simulink library "HIL_GenSet"  (Simulink 7.8)
settings: Solver=ode45  StartTime=0.0  StopTime=10.0  RelTol=1e-3
values from neighbouring files (symbols this model uses):
  Ts = 80e-6    (= 8e-05)    [global_parameters.m]    (also in scopeBuffer.m)
undefined symbols (not defined in the file or in its folder): DiscIntNeverNeededParam, Ts_Power
libraries: simulink x77, powerlib x55, discretizing x28
(part 1 of 9)
settings Model: Creator=RE25624  LastModifiedBy=re25624

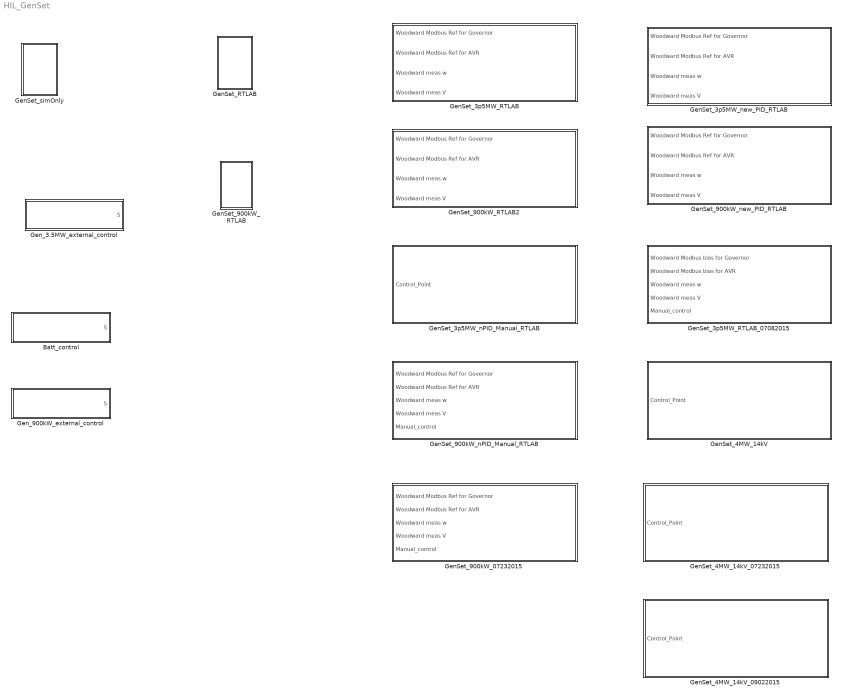
== system HIL_GenSet ==
  Batt_control : Subsystem
  GenSet_3p5MW_RTLAB : Subsystem  mask(Gen-Set with simulated control modes){mode=1 (PQ), set_Pref=0.8, set_Qref=.5, set_vref=1, set_wref=1, enable_gen=1, control_mode=0}
      mask prompts: set_Pref "Active power reference [p.u.]"; set_Qref "Reactive power reference [p.u.]"; set_vref "Terminal voltage reference [p.u.]"; set_wref "Frequency reference [p.u.]"; enable_gen "Enable generator"; control_mode "Control Mode [0 => Sim. 1 => Wood.]"
      mask help:
      | This Gen-Set block allows the user to indicate the control mode of the generator. The available control modes are: (1) PQ, (2) PV, and (3) VF.
      | The input values to the block will be applied according to the selected control mode.
      | For example, if PQ mode is selected, the controller will only work based on P_ref and Q_ref ignoring values of other inputs to the block.
      | *** This model will not interface with a hardware controller ***
      mask StyleString: popup(1 (PQ)|2 (PV)|3 (VF)),edit,edit,edit,edit,popup(1|0),edit
  GenSet_3p5MW_RTLAB_07082015 : Subsystem  mask(Gen-Set (3.5MW) with simulated control modes){control_mode=0}
      mask prompts: control_mode "Control Mode [0 => Sim. 1 => Wood.]"
      mask help:
      | This Gen-Set block (3.5MW) allows the user to indicate the control mode of the generator. The available control modes are: (1) PQ, (2) PV, and (3) VF.
      | The input values to the block will be applied according to the selected control mode.
      | For example, if PQ mode is selected, the controller will only work based on P_ref and Q_ref ignoring values of other inputs to the block.
      | *** This model will not interface with a hardware controller ***
  GenSet_3p5MW_nPID_Manual_RTLAB : Subsystem
      mask Type: Gen-Set (3.5MW) with simulated control modes
      mask Description:
      | This Gen-Set block (3.5MW) allows the user to indicate the control mode of the generator. The available control modes are: (1) PQ, (2) PV, and (3) VF.
      | The input values to the block will be applied according to the selected control mode.
      | For example, if PQ mode is selected, the controller will only work based on P_ref and Q_ref ignoring values of other inputs to the block.
      | *** This model will not interface with a hardware controller ***
      | 
      | Input parameters (as per unit of rated power):
      | P[p.u]: real power
      | Q[p.u]: reactive power
      | V[p.u]: voltage
      | F[p.u]: frequency
      | Mode: (1) PQ, (2) PV, and (3) VF.
  GenSet_3p5MW_new_PID_RTLAB : Subsystem  mask(Gen-Set with simulated control modes){mode=1 (PQ), set_Pref=0.8, set_Qref=0.2, set_vref=1, set_wref=1, enable_gen=1, control_mode=0}
      mask prompts: set_Pref "Active power reference [p.u.]"; set_Qref "Reactive power reference [p.u.]"; set_vref "Terminal voltage reference [p.u.]"; set_wref "Frequency reference [p.u.]"; enable_gen "Enable generator"; control_mode "Control Mode [0 => Sim. 1 => Wood.]"
      mask help:
      | This Gen-Set block allows the user to indicate the control mode of the generator. The available control modes are: (1) PQ, (2) PV, and (3) VF.
      | The input values to the block will be applied according to the selected control mode.
      | For example, if PQ mode is selected, the controller will only work based on P_ref and Q_ref ignoring values of other inputs to the block.
      | *** This model will not interface with a hardware controller ***
      mask StyleString: popup(1 (PQ)|2 (PV)|3 (VF)),edit,edit,edit,edit,popup(1|0),edit
  GenSet_4MW_14kV : Subsystem
      mask Type: Gen-Set (3.5MW) with simulated control modes
      mask Description:
      | This Gen-Set block (3.5MW) allows the user to indicate the control mode of the generator. The available control modes are: (1) PQ, (2) PV, and (3) VF.
      | The input values to the block will be applied according to the selected control mode.
      | For example, if PQ mode is selected, the controller will only work based on P_ref and Q_ref ignoring values of other inputs to the block.
      | *** This model will not interface with a hardware controller ***
      | 
      | Input parameters (as per unit of rated power):
      | P[p.u]: real power
      | Q[p.u]: reactive power
      | V[p.u]: voltage
      | F[p.u]: frequency
      | Mode: (1) PQ, (2) PV, and (3) VF.
  GenSet_4MW_14kV_07232015 : Subsystem
      mask Type: Gen-Set (3.5MW) with simulated control modes
      mask Description:
      | This Gen-Set block (3.5MW) allows the user to indicate the control mode of the generator. The available control modes are: (1) PQ, (2) PV, and (3) VF.
      | The input values to the block will be applied according to the selected control mode.
      | For example, if PQ mode is selected, the controller will only work based on P_ref and Q_ref ignoring values of other inputs to the block.
      | *** This model will not interface with a hardware controller ***
      | 
      | Input parameters (as per unit of rated power):
      | P[p.u]: real power
      | Q[p.u]: reactive power
      | V[p.u]: voltage
      | F[p.u]: frequency
      | Mode: (1) PQ, (2) PV, and (3) VF.
  GenSet_4MW_14kV_09022015 : Subsystem
      mask Type: Gen-Set (3.5MW) with simulated control modes
      mask Description:
      | This Gen-Set block (3.5MW) allows the user to indicate the control mode of the generator. The available control modes are: (1) PQ, (2) PV, and (3) VF.
      | The input values to the block will be applied according to the selected control mode.
      | For example, if PQ mode is selected, the controller will only work based on P_ref and Q_ref ignoring values of other inputs to the block.
      | *** This model will not interface with a hardware controller ***
      | 
      | Input parameters (as per unit of rated power):
      | P[p.u]: real power
      | Q[p.u]: reactive power
      | V[p.u]: voltage
      | F[p.u]: frequency
      | Mode: (1) PQ, (2) PV, and (3) VF.
  GenSet_900kW_07232015 : Subsystem  mask(Gen-Set with simulated control modes){control_mode=0}
      mask prompts: control_mode "Control Mode [0 => Sim. 1 => Wood.]"
      mask help:
      | This Gen-Set block allows the user to indicate the control mode of the generator. The available control modes are: (1) PQ, (2) PV, and (3) VF.
      | The input values to the block will be applied according to the selected control mode.
      | For example, if PQ mode is selected, the controller will only work based on P_ref and Q_ref ignoring values of other inputs to the block.
  GenSet_900kW_RTLAB : Subsystem  mask(Gen-Set with simulated control modes){mode=1 (PQ), set_Pref=0.95, set_Qref=0.85, set_vref=1, set_wref=1, enable_gen=1}
      mask prompts: set_Pref "Active power reference [p.u.]"; set_Qref "Reactive power reference [p.u.]"; set_vref "Terminal voltage reference [p.u.]"; set_wref "Frequency reference [p.u.]"; enable_gen "Enable generator"
      mask help:
      | This Gen-Set block allows the user to indicate the control mode of the generator. The available control modes are: (1) PQ, (2) PV, and (3) VF.
      | The input values to the block will be applied according to the selected control mode.
      | For example, if PQ mode is selected, the controller will only work based on P_ref and Q_ref ignoring values of other inputs to the block.
      | *** This model will not interface with a hardware controller ***
      mask StyleString: popup(1 (PQ)|2 (PV)|3 (VF)),edit,edit,edit,edit,popup(1|0)
  GenSet_900kW_RTLAB2 : Subsystem  mask(Gen-Set with simulated control modes){mode=1 (PQ), set_Pref=0.8, set_Qref=0.2, set_vref=1, set_wref=1, enable_gen=1, control_mode=0}
      mask prompts: set_Pref "Active power reference [p.u.]"; set_Qref "Reactive power reference [p.u.]"; set_vref "Terminal voltage reference [p.u.]"; set_wref "Frequency reference [p.u.]"; enable_gen "Enable generator"; control_mode "Control Mode [0 => Sim. 1 => Wood.]"
      mask help:
      | This Gen-Set block allows the user to indicate the control mode of the generator. The available control modes are: (1) PQ, (2) PV, and (3) VF.
      | The input values to the block will be applied according to the selected control mode.
      | For example, if PQ mode is selected, the controller will only work based on P_ref and Q_ref ignoring values of other inputs to the block.
      | *** This model will not interface with a hardware controller ***
      mask StyleString: popup(1 (PQ)|2 (PV)|3 (VF)),edit,edit,edit,edit,popup(1|0),edit
  GenSet_900kW_nPID_Manual_RTLAB : Subsystem  mask(Gen-Set with simulated control modes){control_mode=0}
      mask prompts: control_mode "Control Mode [0 => Sim. 1 => Wood.]"
      mask help:
      | This Gen-Set block allows the user to indicate the control mode of the generator. The available control modes are: (1) PQ, (2) PV, and (3) VF.
      | The input values to the block will be applied according to the selected control mode.
      | For example, if PQ mode is selected, the controller will only work based on P_ref and Q_ref ignoring values of other inputs to the block.
  GenSet_900kW_new_PID_RTLAB : Subsystem  mask(Gen-Set with simulated control modes){mode=1 (PQ), set_Pref=0.8, set_Qref=0.2, set_vref=1, set_wref=1, enable_gen=1, control_mode=0}
      mask prompts: set_Pref "Active power reference [p.u.]"; set_Qref "Reactive power reference [p.u.]"; set_vref "Terminal voltage reference [p.u.]"; set_wref "Frequency reference [p.u.]"; enable_gen "Enable generator"; control_mode "Control Mode [0 => Sim. 1 => Wood.]"
      mask help:
      | This Gen-Set block allows the user to indicate the control mode of the generator. The available control modes are: (1) PQ, (2) PV, and (3) VF.
      | The input values to the block will be applied according to the selected control mode.
      | For example, if PQ mode is selected, the controller will only work based on P_ref and Q_ref ignoring values of other inputs to the block.
      | *** This model will not interface with a hardware controller ***
      mask StyleString: popup(1 (PQ)|2 (PV)|3 (VF)),edit,edit,edit,edit,popup(1|0),edit
  GenSet_RTLAB : Subsystem  mask(Gen-Set with simulated control modes){mode=3 (VF), set_Pref=0.95, set_Qref=0.85, set_vref=1, set_wref=1, enable_gen=1}
      mask prompts: set_Pref "Active power reference [p.u.]"; set_Qref "Reactive power reference [p.u.]"; set_vref "Terminal voltage reference [p.u.]"; set_wref "Frequency reference [p.u.]"; enable_gen "Enable generator"
      mask help:
      | This Gen-Set block allows the user to indicate the control mode of the generator. The available control modes are: (1) PQ, (2) PV, and (3) VF.
      | The input values to the block will be applied according to the selected control mode.
      | For example, if PQ mode is selected, the controller will only work based on P_ref and Q_ref ignoring values of other inputs to the block.
      | *** This model will not interface with a hardware controller ***
      mask StyleString: popup(1 (PQ)|2 (PV)|3 (VF)),edit,edit,edit,edit,popup(1|0)
  GenSet_simOnly : Subsystem  mask(Gen-Set with simulated control modes){mode=1 (PQ), set_Pref=0.95, set_Qref=0.85, set_vref=1, set_wref=1, enable_gen=1}
      mask prompts: set_Pref "Active power reference [p.u.]"; set_Qref "Reactive power reference [p.u.]"; set_vref "Terminal voltage reference [p.u.]"; set_wref "Frequency reference [p.u.]"; enable_gen "Enable generator"
      mask help:
      | This Gen-Set block allows the user to indicate the control mode of the generator. The available control modes are: (1) PQ, (2) PV, and (3) VF.
      | The input values to the block will be applied according to the selected control mode.
      | For example, if PQ mode is selected, the controller will only work based on P_ref and Q_ref ignoring values of other inputs to the block.
      | *** This model will not interface with a hardware controller ***
      mask StyleString: popup(1 (PQ)|2 (PV)|3 (VF)),edit,edit,edit,edit,popup(1|0)
  Gen_3.5MW_external_control : Subsystem
  Gen_900kW_external_control : Subsystem

== system HIL_GenSet/Batt_control ==
  Bus Creator : BusCreator  Inputs=3
  DONOTCHANGE : Constant
  Enable : Constant  Value=0
  kW : simulink/Math Operations/Slider Gain  low=1  gain=500  high=1000
  kvar : simulink/Math Operations/Slider Gain  low=1  gain=200  high=500
  S : Outport
  wires:
  kW/1 -> Bus Creator/2  "kW"
  kvar/1 -> Bus Creator/1  "kvar"
  Bus Creator/1 -> S/1
  DONOTCHANGE/1 -> kvar/1, kW/1
  Enable/1 -> Bus Creator/3

== system HIL_GenSet/GenSet_3p5MW_RTLAB ==
  note: Modbus Register for the values.
  note: Voltage and Currents of Generator.
      | This will be outputs of the HIL Unit
      | and inputs to the device controller.
      | Need to T off lines if use here.
  Woodward Modbus Ref for Governor : Inport
  Woodward Modbus Ref for AVR : Inport  Port=2
  Woodward meas w : Inport  Port=3
  Woodward meas V : Inport  Port=4
  60kW Generator with  Primary Controllers : Subsystem
  Demux : Demux  Outputs=2
  DocBlock : simulink/Model-Wide Utilities/DocBlock  DocumentType=Text
  Enable_generator : Constant  Value=enable_gen
  Interface between Woodward Controller and simated generator : Subsystem
  Scope : Scope  NumInputPorts=2
      settings: YMin=0.995~0.925  YMax=1.05~1.05
  Simulated Generator Controller : Subsystem
  Switch : Switch  Threshold=0.5
  control mode 1 for Woodward 0 for simulation 1 : Constant  Value=control_mode
  A : PMIOPort  Port=1  Side=Right
  B : PMIOPort  Port=2  Side=Right
  C : PMIOPort  Port=3  Side=Right
  tag scope: cntrl_mode=global, gen_m=global
  wires:
  Simulated Generator Controller/1("wref, Vref") -> Switch/3  "simulated"
  Enable_generator/1 -> 60kW Generator with  Primary Controllers/3(Enable)
  60kW Generator with  Primary Controllers/1(m) -> [gen_m]
  Demux/1 -> 60kW Generator with  Primary Controllers/1(wref), Scope/1  "w_ref"
  Demux/2 -> 60kW Generator with  Primary Controllers/2(Vtref), Scope/2  "v_ref"
  Interface between Woodward Controller and simated generator/1(wref,Vref) -> Switch/1
  Switch/1 -> Demux/1
  control mode 1 for Woodward 0 for simulation 1/1 -> [cntrl_mode]
  [cntrl_mode] -> Switch/2
  Woodward Modbus Ref for Governor/1 -> Interface between Woodward Controller and simated generator/1(Woodward for wref)
  Woodward Modbus Ref for AVR/1 -> Interface between Woodward Controller and simated generator/2(Woodward for Vref)
  Woodward meas w/1 -> 60kW Generator with  Primary Controllers/4(w_meas_Woodward)
  Woodward meas V/1 -> 60kW Generator with  Primary Controllers/5(V_meas_Woodward)
  connections:
  A/RConn1 -- 60kW Generator with  Primary Controllers/RConn1
  60kW Generator with  Primary Controllers/RConn2 -- B/RConn1
  C/RConn1 -- 60kW Generator with  Primary Controllers/RConn3

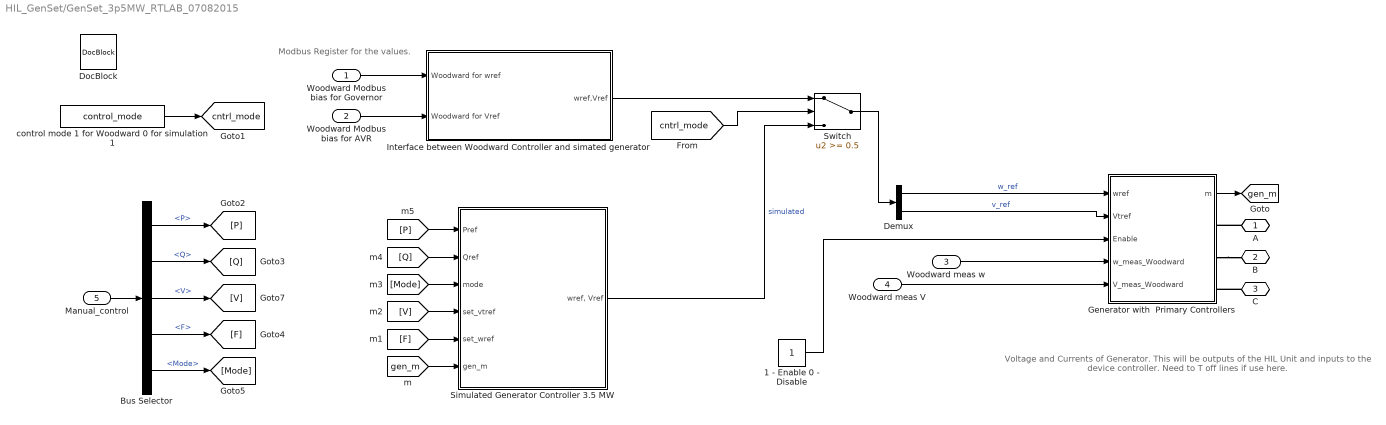
== system HIL_GenSet/GenSet_3p5MW_RTLAB_07082015 ==
  note: Modbus Register for the values.
  note: Voltage and Currents of Generator.
      | This will be outputs of the HIL Unit
      | and inputs to the device controller.
      | Need to T off lines if use here.
  Woodward Modbus bias for Governor : Inport
  Woodward Modbus bias for AVR : Inport  Port=2
  Woodward meas w : Inport  Port=3
  Woodward meas V : Inport  Port=4
  Manual_control : Inport  Port=5
  1 - Enable 0 - Disable : Constant
  Bus Selector : BusSelector  OutputSignals=P,Q,V,F,Mode
  Demux : Demux  Outputs=2
  DocBlock : simulink/Model-Wide Utilities/DocBlock  DocumentType=Text
  Generator with  Primary Controllers : Subsystem
  Interface between Woodward Controller and simated generator : Subsystem
  Simulated Generator Controller 3.5 MW : Subsystem
  Switch : Switch  Threshold=0.5
  control mode 1 for Woodward 0 for simulation 1 : Constant  Value=control_mode
  A : PMIOPort  Port=1  Side=Right
  B : PMIOPort  Port=2  Side=Right
  C : PMIOPort  Port=3  Side=Right
  tag scope: cntrl_mode=global, gen_m=global
  wires:
  1 - Enable 0 - Disable/1 -> Generator with  Primary Controllers/3(Enable)
  [gen_m] -> Simulated Generator Controller 3.5 MW/6(gen_m)
  [P] -> Simulated Generator Controller 3.5 MW/1(Pref)
  [Q] -> Simulated Generator Controller 3.5 MW/2(Qref)
  [Mode] -> Simulated Generator Controller 3.5 MW/3(mode)
  [V] -> Simulated Generator Controller 3.5 MW/4(set_vtref)
  [F] -> Simulated Generator Controller 3.5 MW/5(set_wref)
  Manual_control/1 -> Bus Selector/1
  Bus Selector/1 -> [P]  "<P>"
  Bus Selector/2 -> [Q]  "<Q>"
  Bus Selector/3 -> [V]  "<V>"
  Bus Selector/4 -> [F]  "<F>"
  Bus Selector/5 -> [Mode]  "<Mode>"
  Simulated Generator Controller 3.5 MW/1("wref, Vref") -> Switch/3  "simulated"
  Generator with  Primary Controllers/1(m) -> [gen_m]
  Demux/1 -> Generator with  Primary Controllers/1(wref)  "w_ref"
  Demux/2 -> Generator with  Primary Controllers/2(Vtref)  "v_ref"
  Interface between Woodward Controller and simated generator/1(wref,Vref) -> Switch/1
  Switch/1 -> Demux/1
  control mode 1 for Woodward 0 for simulation 1/1 -> [cntrl_mode]
  [cntrl_mode] -> Switch/2
  Woodward Modbus bias for Governor/1 -> Interface between Woodward Controller and simated generator/1(Woodward for wref)
  Woodward Modbus bias for AVR/1 -> Interface between Woodward Controller and simated generator/2(Woodward for Vref)
  Woodward meas w/1 -> Generator with  Primary Controllers/4(w_meas_Woodward)
  Woodward meas V/1 -> Generator with  Primary Controllers/5(V_meas_Woodward)
  connections:
  A/RConn1 -- Generator with  Primary Controllers/RConn1
  Generator with  Primary Controllers/RConn2 -- B/RConn1
  C/RConn1 -- Generator with  Primary Controllers/RConn3

== system HIL_GenSet/GenSet_3p5MW_nPID_Manual_RTLAB ==
  note: Voltage and Currents of Generator.
      | This will be outputs of the HIL Unit
      | and inputs to the device controller.
      | Need to T off lines if use here.
  Control_Point : Inport
  1 - Enable 0 - Disable : Constant
  Bus Selector : BusSelector  OutputSignals=P,Q,V,F,Mode
  Demux : Demux  Outputs=2
  DocBlock : simulink/Model-Wide Utilities/DocBlock  DocumentType=Text
  Generator with  Primary Controllers : Subsystem
  Simulated Generator Controller 3.5 MW : Subsystem
  A : PMIOPort  Port=1  Side=Right
  B : PMIOPort  Port=2  Side=Right
  C : PMIOPort  Port=3  Side=Right
  tag scope: gen_m=global
  wires:
  Simulated Generator Controller 3.5 MW/1("wref, Vref") -> Demux/1  "simulated"
  1 - Enable 0 - Disable/1 -> Generator with  Primary Controllers/3(Enable)
  [gen_m] -> Simulated Generator Controller 3.5 MW/6(gen_m)
  [P] -> Simulated Generator Controller 3.5 MW/1(Pref)
  [Q] -> Simulated Generator Controller 3.5 MW/2(Qref)
  [Mode] -> Simulated Generator Controller 3.5 MW/3(mode)
  [V] -> Simulated Generator Controller 3.5 MW/4(set_vtref)
  [F] -> Simulated Generator Controller 3.5 MW/5(set_wref)
  Control_Point/1 -> Bus Selector/1
  Bus Selector/1 -> [P]  "<P>"
  Bus Selector/2 -> [Q]  "<Q>"
  Bus Selector/3 -> [V]  "<V>"
  Bus Selector/4 -> [F]  "<F>"
  Bus Selector/5 -> [Mode]  "<Mode>"
  Generator with  Primary Controllers/1(m) -> [gen_m]
  Demux/1 -> Generator with  Primary Controllers/1(wref)  "w_ref"
  Demux/2 -> Generator with  Primary Controllers/2(Vtref)  "v_ref"
  connections:
  A/RConn1 -- Generator with  Primary Controllers/RConn1
  Generator with  Primary Controllers/RConn2 -- B/RConn1
  C/RConn1 -- Generator with  Primary Controllers/RConn3

== system HIL_GenSet/GenSet_3p5MW_new_PID_RTLAB ==
  note: Modbus Register for the values.
  note: Voltage and Currents of Generator.
      | This will be outputs of the HIL Unit
      | and inputs to the device controller.
      | Need to T off lines if use here.
  Woodward Modbus Ref for Governor : Inport
  Woodward Modbus Ref for AVR : Inport  Port=2
  Woodward meas w : Inport  Port=3
  Woodward meas V : Inport  Port=4
  60kW Generator with  Primary Controllers : Subsystem
  Demux : Demux  Outputs=2
  DocBlock : simulink/Model-Wide Utilities/DocBlock  DocumentType=Text
  Enable_generator : Constant  Value=enable_gen
  Interface between Woodward Controller and simated generator : Subsystem
  Scope : Scope  NumInputPorts=2
      settings: YMin=0.995~0.925  YMax=1.05~1.05
  Simulated Generator Controller : Subsystem
  Switch : Switch  Threshold=0.5
  control mode 1 for Woodward 0 for simulation 1 : Constant  Value=control_mode
  A : PMIOPort  Port=1  Side=Right
  B : PMIOPort  Port=2  Side=Right
  C : PMIOPort  Port=3  Side=Right
  tag scope: cntrl_mode=global, gen_m=global
  wires:
  Simulated Generator Controller/1("wref, Vref") -> Switch/3  "simulated"
  Enable_generator/1 -> 60kW Generator with  Primary Controllers/3(Enable)
  60kW Generator with  Primary Controllers/1(m) -> [gen_m]
  Demux/1 -> 60kW Generator with  Primary Controllers/1(wref), Scope/1  "w_ref"
  Demux/2 -> 60kW Generator with  Primary Controllers/2(Vtref), Scope/2  "v_ref"
  Interface between Woodward Controller and simated generator/1(wref,Vref) -> Switch/1
  Switch/1 -> Demux/1
  control mode 1 for Woodward 0 for simulation 1/1 -> [cntrl_mode]
  [cntrl_mode] -> Switch/2
  Woodward Modbus Ref for Governor/1 -> Interface between Woodward Controller and simated generator/1(Woodward for wref)
  Woodward Modbus Ref for AVR/1 -> Interface between Woodward Controller and simated generator/2(Woodward for Vref)
  Woodward meas w/1 -> 60kW Generator with  Primary Controllers/4(w_meas_Woodward)
  Woodward meas V/1 -> 60kW Generator with  Primary Controllers/5(V_meas_Woodward)
  connections:
  A/RConn1 -- 60kW Generator with  Primary Controllers/RConn1
  60kW Generator with  Primary Controllers/RConn2 -- B/RConn1
  C/RConn1 -- 60kW Generator with  Primary Controllers/RConn3

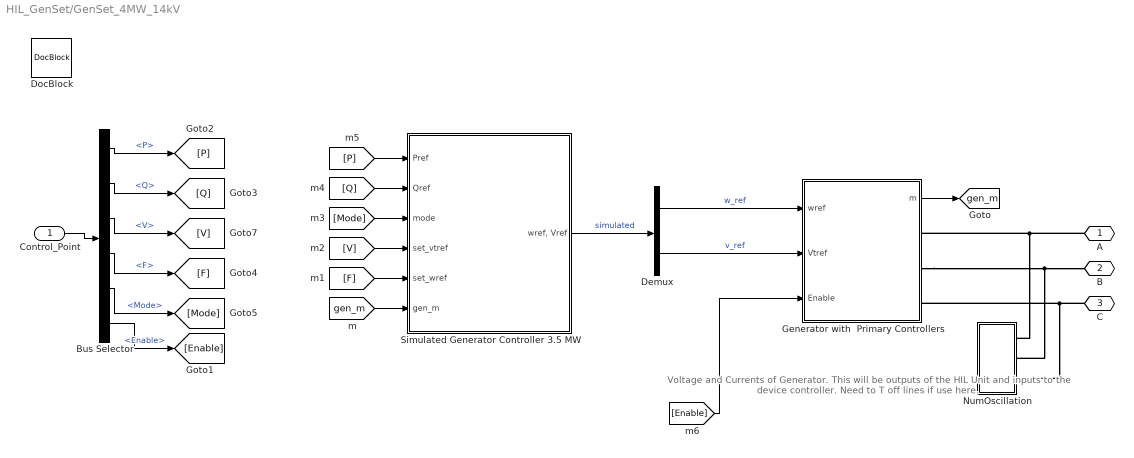
== system HIL_GenSet/GenSet_4MW_14kV ==
  note: Voltage and Currents of Generator.
      | This will be outputs of the HIL Unit
      | and inputs to the device controller.
      | Need to T off lines if use here.
  Control_Point : Inport
  Bus Selector : BusSelector  OutputSignals=P,Q,V,F,Mode,Enable
  Demux : Demux  Outputs=2
  DocBlock : simulink/Model-Wide Utilities/DocBlock  DocumentType=Text
  Generator with  Primary Controllers : Subsystem
  NumOscillation : Subsystem
  Simulated Generator Controller 3.5 MW : Subsystem
  A : PMIOPort  Port=1  Side=Right
  B : PMIOPort  Port=2  Side=Right
  C : PMIOPort  Port=3  Side=Right
  tag scope: gen_m=global
  wires:
  Simulated Generator Controller 3.5 MW/1("wref, Vref") -> Demux/1  "simulated"
  [Enable] -> Generator with  Primary Controllers/3(Enable)
  [gen_m] -> Simulated Generator Controller 3.5 MW/6(gen_m)
  [P] -> Simulated Generator Controller 3.5 MW/1(Pref)
  [Q] -> Simulated Generator Controller 3.5 MW/2(Qref)
  [Mode] -> Simulated Generator Controller 3.5 MW/3(mode)
  [V] -> Simulated Generator Controller 3.5 MW/4(set_vtref)
  [F] -> Simulated Generator Controller 3.5 MW/5(set_wref)
  Control_Point/1 -> Bus Selector/1
  Bus Selector/1 -> [P]  "<P>"
  Bus Selector/2 -> [Q]  "<Q>"
  Bus Selector/3 -> [V]  "<V>"
  Bus Selector/4 -> [F]  "<F>"
  Bus Selector/5 -> [Mode]  "<Mode>"
  Generator with  Primary Controllers/1(m) -> [gen_m]
  Demux/1 -> Generator with  Primary Controllers/1(wref)  "w_ref"
  Demux/2 -> Generator with  Primary Controllers/2(Vtref)  "v_ref"
  Bus Selector/6 -> [Enable]  "<Enable>"
  connections:
  A/RConn1 -- Generator with  Primary Controllers/RConn1 -- NumOscillation/LConn1
  Generator with  Primary Controllers/RConn2 -- B/RConn1 -- NumOscillation/LConn2
  C/RConn1 -- Generator with  Primary Controllers/RConn3 -- NumOscillation/LConn3

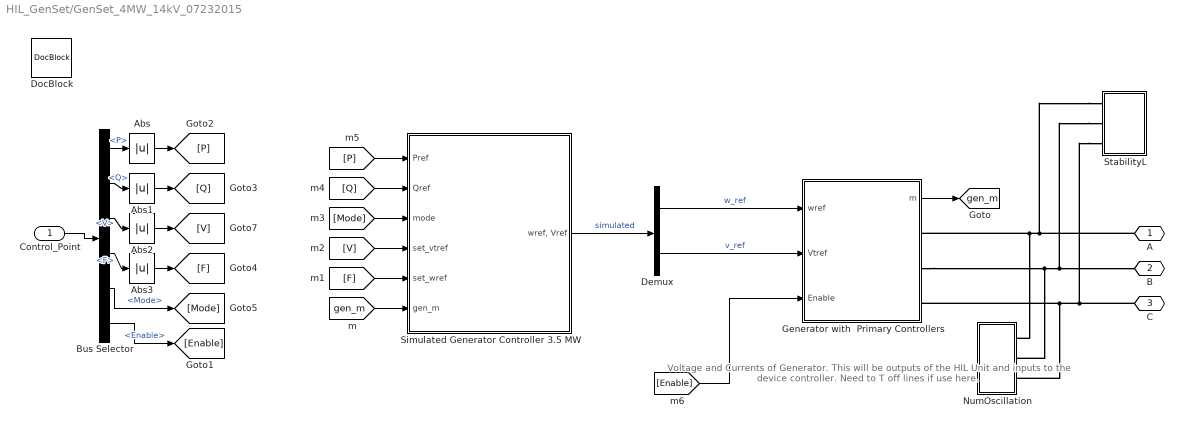
== system HIL_GenSet/GenSet_4MW_14kV_07232015 ==
  note: Voltage and Currents of Generator.
      | This will be outputs of the HIL Unit
      | and inputs to the device controller.
      | Need to T off lines if use here.
  Control_Point : Inport
  Abs{,1..3} (4 alike) : Abs
  Bus Selector : BusSelector  OutputSignals=P,Q,V,F,Mode,Enable
  Demux : Demux  Outputs=2
  DocBlock : simulink/Model-Wide Utilities/DocBlock  DocumentType=Text
  Generator with  Primary Controllers : Subsystem
  NumOscillation : Subsystem
  Simulated Generator Controller 3.5 MW : Subsystem
  StabilityL : Subsystem  mask{v=13800, kVA=150, pf=1}
  A : PMIOPort  Port=1  Side=Right
  B : PMIOPort  Port=2  Side=Right
  C : PMIOPort  Port=3  Side=Right
  tag scope: gen_m=global
  wires:
  Simulated Generator Controller 3.5 MW/1("wref, Vref") -> Demux/1  "simulated"
  [Enable] -> Generator with  Primary Controllers/3(Enable)
  [gen_m] -> Simulated Generator Controller 3.5 MW/6(gen_m)
  [P] -> Simulated Generator Controller 3.5 MW/1(Pref)
  [Q] -> Simulated Generator Controller 3.5 MW/2(Qref)
  [Mode] -> Simulated Generator Controller 3.5 MW/3(mode)
  [V] -> Simulated Generator Controller 3.5 MW/4(set_vtref)
  [F] -> Simulated Generator Controller 3.5 MW/5(set_wref)
  Control_Point/1 -> Bus Selector/1
  Bus Selector/1 -> Abs/1  "<P>"
  Bus Selector/2 -> Abs1/1  "<Q>"
  Bus Selector/3 -> Abs2/1  "<V>"
  Bus Selector/4 -> Abs3/1  "<F>"
  Bus Selector/5 -> [Mode]  "<Mode>"
  Generator with  Primary Controllers/1(m) -> [gen_m]
  Demux/1 -> Generator with  Primary Controllers/1(wref)  "w_ref"
  Demux/2 -> Generator with  Primary Controllers/2(Vtref)  "v_ref"
  Bus Selector/6 -> [Enable]  "<Enable>"
  Abs/1 -> [P]
  Abs1/1 -> [Q]
  Abs2/1 -> [V]
  Abs3/1 -> [F]
  connections:
  StabilityL/LConn1 -- Generator with  Primary Controllers/RConn1 -- NumOscillation/LConn1 -- A/RConn1
  StabilityL/LConn2 -- B/RConn1 -- Generator with  Primary Controllers/RConn2 -- NumOscillation/LConn2
  StabilityL/LConn3 -- Generator with  Primary Controllers/RConn3 -- NumOscillation/LConn3 -- C/RConn1

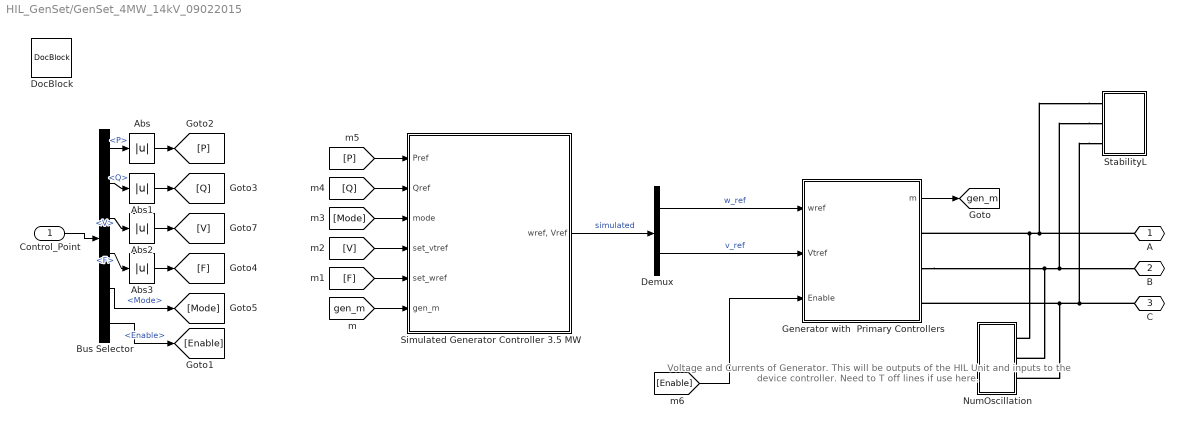
== system HIL_GenSet/GenSet_4MW_14kV_09022015 ==
  note: Voltage and Currents of Generator.
      | This will be outputs of the HIL Unit
      | and inputs to the device controller.
      | Need to T off lines if use here.
  Control_Point : Inport
  Abs{,1..3} (4 alike) : Abs
  Bus Selector : BusSelector  OutputSignals=P,Q,V,F,Mode,Enable
  Demux : Demux  Outputs=2
  DocBlock : simulink/Model-Wide Utilities/DocBlock  DocumentType=Text
  Generator with  Primary Controllers : Subsystem
  NumOscillation : Subsystem
  Simulated Generator Controller 3.5 MW : Subsystem
  StabilityL : Subsystem  mask{v=13800, kVA=300, pf=1}
  A : PMIOPort  Port=1  Side=Right
  B : PMIOPort  Port=2  Side=Right
  C : PMIOPort  Port=3  Side=Right
  tag scope: gen_m=global
  wires:
  Simulated Generator Controller 3.5 MW/1("wref, Vref") -> Demux/1  "simulated"
  [Enable] -> Generator with  Primary Controllers/3(Enable)
  [gen_m] -> Simulated Generator Controller 3.5 MW/6(gen_m)
  [P] -> Simulated Generator Controller 3.5 MW/1(Pref)
  [Q] -> Simulated Generator Controller 3.5 MW/2(Qref)
  [Mode] -> Simulated Generator Controller 3.5 MW/3(mode)
  [V] -> Simulated Generator Controller 3.5 MW/4(set_vtref)
  [F] -> Simulated Generator Controller 3.5 MW/5(set_wref)
  Control_Point/1 -> Bus Selector/1
  Bus Selector/1 -> Abs/1  "<P>"
  Bus Selector/2 -> Abs1/1  "<Q>"
  Bus Selector/3 -> Abs2/1  "<V>"
  Bus Selector/4 -> Abs3/1  "<F>"
  Bus Selector/5 -> [Mode]  "<Mode>"
  Generator with  Primary Controllers/1(m) -> [gen_m]
  Demux/1 -> Generator with  Primary Controllers/1(wref)  "w_ref"
  Demux/2 -> Generator with  Primary Controllers/2(Vtref)  "v_ref"
  Bus Selector/6 -> [Enable]  "<Enable>"
  Abs/1 -> [P]
  Abs1/1 -> [Q]
  Abs2/1 -> [V]
  Abs3/1 -> [F]
  connections:
  StabilityL/LConn1 -- Generator with  Primary Controllers/RConn1 -- NumOscillation/LConn1 -- A/RConn1
  StabilityL/LConn2 -- B/RConn1 -- Generator with  Primary Controllers/RConn2 -- NumOscillation/LConn2
  StabilityL/LConn3 -- Generator with  Primary Controllers/RConn3 -- NumOscillation/LConn3 -- C/RConn1

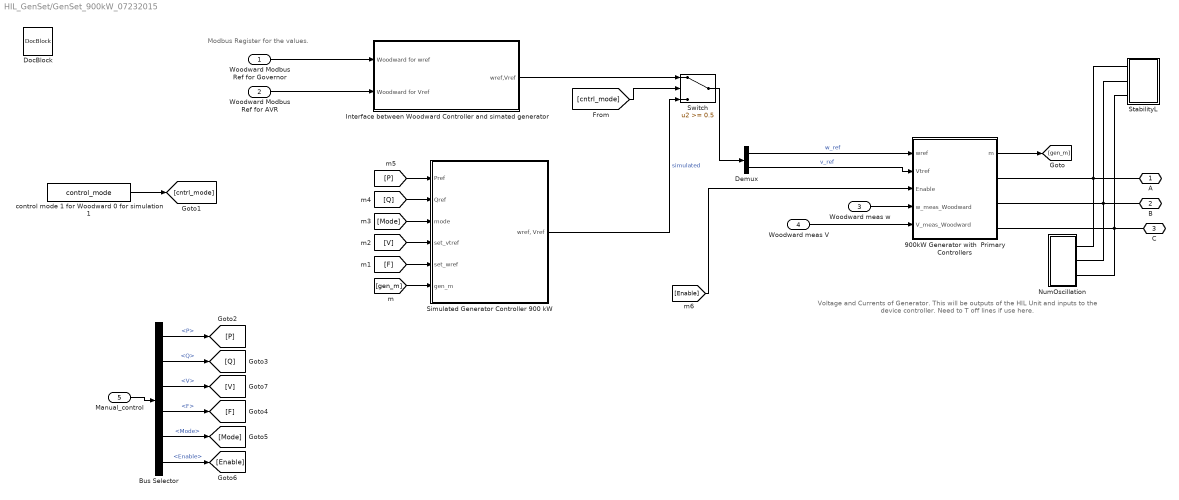
== system HIL_GenSet/GenSet_900kW_07232015 ==
  note: Modbus Register for the values.
  note: Voltage and Currents of Generator.
      | This will be outputs of the HIL Unit
      | and inputs to the device controller.
      | Need to T off lines if use here.
  Woodward Modbus Ref for Governor : Inport
  Woodward Modbus Ref for AVR : Inport  Port=2
  Woodward meas w : Inport  Port=3
  Woodward meas V : Inport  Port=4
  Manual_control : Inport  Port=5
  900kW Generator with  Primary Controllers : Subsystem
  Bus Selector : BusSelector  OutputSignals=P,Q,V,F,Mode,Enable
  Demux : Demux  Outputs=2
  DocBlock : simulink/Model-Wide Utilities/DocBlock  DocumentType=Text
  Interface between Woodward Controller and simated generator : Subsystem
  NumOscillation : Subsystem
  Simulated Generator Controller 900 kW : Subsystem
  StabilityL : Subsystem  mask{v=460, kVA=50, pf=1}
  Switch : Switch  Threshold=0.5
  control mode 1 for Woodward 0 for simulation 1 : Constant  Value=control_mode
  A : PMIOPort  Port=1  Side=Right
  B : PMIOPort  Port=2  Side=Right
  C : PMIOPort  Port=3  Side=Right
  wires:
  [F] -> Simulated Generator Controller 900 kW/5(set_wref)
  [V] -> Simulated Generator Controller 900 kW/4(set_vtref)
  [Mode] -> Simulated Generator Controller 900 kW/3(mode)
  [Q] -> Simulated Generator Controller 900 kW/2(Qref)
  [P] -> Simulated Generator Controller 900 kW/1(Pref)
  [gen_m] -> Simulated Generator Controller 900 kW/6(gen_m)
  Bus Selector/5 -> [Mode]  "<Mode>"
  Bus Selector/4 -> [F]  "<F>"
  Bus Selector/3 -> [V]  "<V>"
  Bus Selector/2 -> [Q]  "<Q>"
  Bus Selector/1 -> [P]  "<P>"
  Manual_control/1 -> Bus Selector/1
  Simulated Generator Controller 900 kW/1("wref, Vref") -> Switch/3  "simulated"
  [Enable] -> 900kW Generator with  Primary Controllers/3(Enable)
  900kW Generator with  Primary Controllers/1(m) -> [gen_m]
  Demux/1 -> 900kW Generator with  Primary Controllers/1(wref)  "w_ref"
  Demux/2 -> 900kW Generator with  Primary Controllers/2(Vtref)  "v_ref"
  Interface between Woodward Controller and simated generator/1(wref,Vref) -> Switch/1
  Switch/1 -> Demux/1
  control mode 1 for Woodward 0 for simulation 1/1 -> [cntrl_mode]
  [cntrl_mode] -> Switch/2
  Woodward Modbus Ref for Governor/1 -> Interface between Woodward Controller and simated generator/1(Woodward for wref)
  Woodward Modbus Ref for AVR/1 -> Interface between Woodward Controller and simated generator/2(Woodward for Vref)
  Woodward meas w/1 -> 900kW Generator with  Primary Controllers/4(w_meas_Woodward)
  Woodward meas V/1 -> 900kW Generator with  Primary Controllers/5(V_meas_Woodward)
  Bus Selector/6 -> [Enable]  "<Enable>"
  connections:
  StabilityL/LConn1 -- A/RConn1 -- 900kW Generator with  Primary Controllers/RConn1 -- NumOscillation/LConn1
  StabilityL/LConn2 -- 900kW Generator with  Primary Controllers/RConn2 -- B/RConn1 -- NumOscillation/LConn2
  StabilityL/LConn3 -- C/RConn1 -- 900kW Generator with  Primary Controllers/RConn3 -- NumOscillation/LConn3

== system HIL_GenSet/GenSet_900kW_RTLAB ==
  Bus Selector1 : BusSelector  OutputSignals="Output active power   Peo (pu),Output reactive power  Qeo (pu)"
  Demux : Demux  Outputs=2
  Enable_generator : Constant  Value=enable_gen
  Generator with  Primary Controllers1 : Subsystem
  Multiport Switch : MultiPortSwitch  zeroidx=off
  Mux1 : Mux  Inputs=2
  Mux2 : Mux  Inputs=2
  Mux3 : Mux  Inputs=2
  PQ control : Subsystem
  PV control : Subsystem
  Pref : Constant  Value=set_Pref
  Qref : Constant  Value=set_Qref
  mode (1-3) : Constant  Value=mode
  set_vtref : Constant  Value=set_vref
  set_wref : Constant  Value=set_wref
  A : PMIOPort  Port=1  Side=Right
  B : PMIOPort  Port=2  Side=Right
  C : PMIOPort  Port=3  Side=Right
  wires:
  Generator with  Primary Controllers1/1(m) -> [gen_m]
  Enable_generator/1 -> Generator with  Primary Controllers1/3(Enable)
  mode (1-3)/1 -> Multiport Switch/1
  Qref/1 -> PQ control/3(Q_ref (pu))
  set_wref/1 -> Mux3/1
  Bus Selector1/2 -> PQ control/4(Q (pu))  "<Output reactive power  Qeo (pu)>"
  Pref/1 -> PV control/1(P_ref (pu)), PQ control/1(P_ref (pu))
  Mux3/1 -> Multiport Switch/4
  Mux2/1 -> Multiport Switch/3
  Mux1/1 -> Multiport Switch/2
  set_vtref/1 -> Mux3/2, Mux2/2
  Demux/2 -> Generator with  Primary Controllers1/2(Vtref)  "v_ref"
  Demux/1 -> Generator with  Primary Controllers1/1(wref)  "w_ref"
  Multiport Switch/1 -> Demux/1
  PV control/1(w_ref (pu)) -> Mux2/1
  PQ control/2(V_ref (pu)) -> Mux1/2
  PQ control/1(w_ref (pu)) -> Mux1/1
  [gen_m] -> Bus Selector1/1
  Bus Selector1/1 -> PV control/2(P (pu)), PQ control/2(P (pu))  "<Output active power   Peo (pu)>"
  connections:
  C/RConn1 -- Generator with  Primary Controllers1/RConn3
  B/RConn1 -- Generator with  Primary Controllers1/RConn2
  A/RConn1 -- Generator with  Primary Controllers1/RConn1

== system HIL_GenSet/GenSet_900kW_RTLAB2 ==
  note: Modbus Register for the values.
  note: Voltage and Currents of Generator.
      | This will be outputs of the HIL Unit
      | and inputs to the device controller.
      | Need to T off lines if use here.
  Woodward Modbus Ref for Governor : Inport
  Woodward Modbus Ref for AVR : Inport  Port=2
  Woodward meas w : Inport  Port=3
  Woodward meas V : Inport  Port=4
  60kW Generator with  Primary Controllers : Subsystem
  Demux : Demux  Outputs=2
  DocBlock : simulink/Model-Wide Utilities/DocBlock  DocumentType=Text
  Enable_generator : Constant  Value=enable_gen
  Interface between Woodward Controller and simated generator : Subsystem
  Scope : Scope  NumInputPorts=2
      settings: YMin=0.995~0.925  YMax=1.05~1.05
  Simulated Generator Controller : Subsystem
  Switch : Switch  Threshold=0.5
  control mode 1 for Woodward 0 for simulation 1 : Constant  Value=control_mode
  A : PMIOPort  Port=1  Side=Right
  B : PMIOPort  Port=2  Side=Right
  C : PMIOPort  Port=3  Side=Right
  tag scope: cntrl_mode=global, gen_m=global
  wires:
  Simulated Generator Controller/1("wref, Vref") -> Switch/3  "simulated"
  Enable_generator/1 -> 60kW Generator with  Primary Controllers/3(Enable)
  60kW Generator with  Primary Controllers/1(m) -> [gen_m]
  Demux/1 -> 60kW Generator with  Primary Controllers/1(wref), Scope/1  "w_ref"
  Demux/2 -> 60kW Generator with  Primary Controllers/2(Vtref), Scope/2  "v_ref"
  Interface between Woodward Controller and simated generator/1(wref,Vref) -> Switch/1
  Switch/1 -> Demux/1
  control mode 1 for Woodward 0 for simulation 1/1 -> [cntrl_mode]
  [cntrl_mode] -> Switch/2
  Woodward Modbus Ref for Governor/1 -> Interface between Woodward Controller and simated generator/1(Woodward for wref)
  Woodward Modbus Ref for AVR/1 -> Interface between Woodward Controller and simated generator/2(Woodward for Vref)
  Woodward meas w/1 -> 60kW Generator with  Primary Controllers/4(w_meas_Woodward)
  Woodward meas V/1 -> 60kW Generator with  Primary Controllers/5(V_meas_Woodward)
  connections:
  A/RConn1 -- 60kW Generator with  Primary Controllers/RConn1
  60kW Generator with  Primary Controllers/RConn2 -- B/RConn1
  C/RConn1 -- 60kW Generator with  Primary Controllers/RConn3

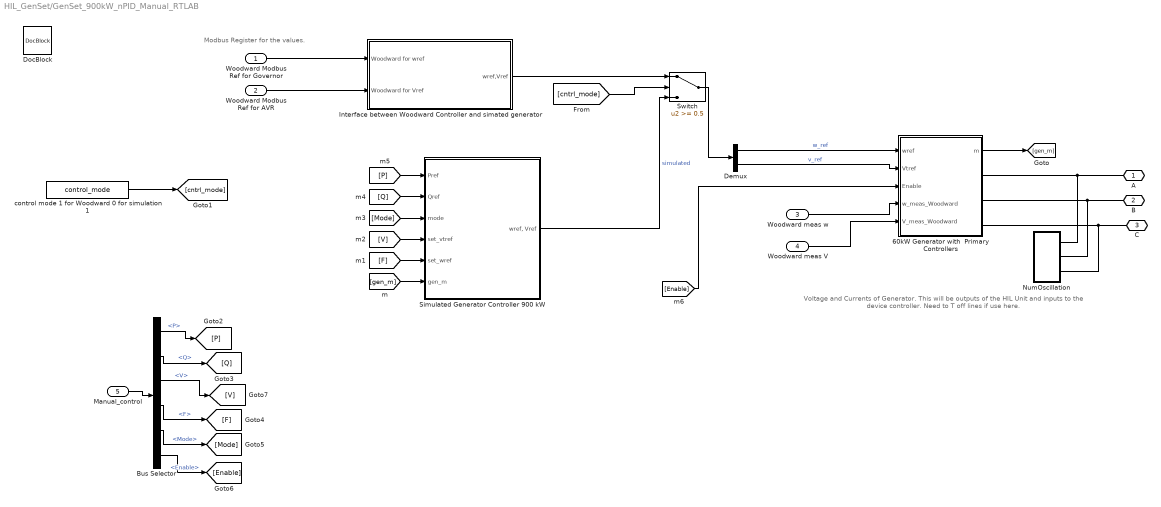
== system HIL_GenSet/GenSet_900kW_nPID_Manual_RTLAB ==
  note: Modbus Register for the values.
  note: Voltage and Currents of Generator.
      | This will be outputs of the HIL Unit
      | and inputs to the device controller.
      | Need to T off lines if use here.
  Woodward Modbus Ref for Governor : Inport
  Woodward Modbus Ref for AVR : Inport  Port=2
  Woodward meas w : Inport  Port=3
  Woodward meas V : Inport  Port=4
  Manual_control : Inport  Port=5
  60kW Generator with  Primary Controllers : Subsystem
  Bus Selector : BusSelector  OutputSignals=P,Q,V,F,Mode,Enable
  Demux : Demux  Outputs=2
  DocBlock : simulink/Model-Wide Utilities/DocBlock  DocumentType=Text
  Interface between Woodward Controller and simated generator : Subsystem
  NumOscillation : Subsystem
  Simulated Generator Controller 900 kW : Subsystem
  Switch : Switch  Threshold=0.5
  control mode 1 for Woodward 0 for simulation 1 : Constant  Value=control_mode
  A : PMIOPort  Port=1  Side=Right
  B : PMIOPort  Port=2  Side=Right
  C : PMIOPort  Port=3  Side=Right
  wires:
  [F] -> Simulated Generator Controller 900 kW/5(set_wref)
  [V] -> Simulated Generator Controller 900 kW/4(set_vtref)
  [Mode] -> Simulated Generator Controller 900 kW/3(mode)
  [Q] -> Simulated Generator Controller 900 kW/2(Qref)
  [P] -> Simulated Generator Controller 900 kW/1(Pref)
  [gen_m] -> Simulated Generator Controller 900 kW/6(gen_m)
  Bus Selector/5 -> [Mode]  "<Mode>"
  Bus Selector/4 -> [F]  "<F>"
  Bus Selector/3 -> [V]  "<V>"
  Bus Selector/2 -> [Q]  "<Q>"
  Bus Selector/1 -> [P]  "<P>"
  Manual_control/1 -> Bus Selector/1
  Simulated Generator Controller 900 kW/1("wref, Vref") -> Switch/3  "simulated"
  [Enable] -> 60kW Generator with  Primary Controllers/3(Enable)
  60kW Generator with  Primary Controllers/1(m) -> [gen_m]
  Demux/1 -> 60kW Generator with  Primary Controllers/1(wref)  "w_ref"
  Demux/2 -> 60kW Generator with  Primary Controllers/2(Vtref)  "v_ref"
  Interface between Woodward Controller and simated generator/1(wref,Vref) -> Switch/1
  Switch/1 -> Demux/1
  control mode 1 for Woodward 0 for simulation 1/1 -> [cntrl_mode]
  [cntrl_mode] -> Switch/2
  Woodward Modbus Ref for Governor/1 -> Interface between Woodward Controller and simated generator/1(Woodward for wref)
  Woodward Modbus Ref for AVR/1 -> Interface between Woodward Controller and simated generator/2(Woodward for Vref)
  Woodward meas w/1 -> 60kW Generator with  Primary Controllers/4(w_meas_Woodward)
  Woodward meas V/1 -> 60kW Generator with  Primary Controllers/5(V_meas_Woodward)
  Bus Selector/6 -> [Enable]  "<Enable>"
  connections:
  A/RConn1 -- 60kW Generator with  Primary Controllers/RConn1 -- NumOscillation/LConn1
  60kW Generator with  Primary Controllers/RConn2 -- B/RConn1 -- NumOscillation/LConn2
  C/RConn1 -- 60kW Generator with  Primary Controllers/RConn3 -- NumOscillation/LConn3

== system HIL_GenSet/GenSet_900kW_new_PID_RTLAB ==
  note: Modbus Register for the values.
  note: Voltage and Currents of Generator.
      | This will be outputs of the HIL Unit
      | and inputs to the device controller.
      | Need to T off lines if use here.
  Woodward Modbus Ref for Governor : Inport
  Woodward Modbus Ref for AVR : Inport  Port=2
  Woodward meas w : Inport  Port=3
  Woodward meas V : Inport  Port=4
  60kW Generator with  Primary Controllers : Subsystem
  Demux : Demux  Outputs=2
  DocBlock : simulink/Model-Wide Utilities/DocBlock  DocumentType=Text
  Enable_generator : Constant  Value=enable_gen
  Interface between Woodward Controller and simated generator : Subsystem
  Scope : Scope  NumInputPorts=2
      settings: YMin=0.995~0.925  YMax=1.05~1.05
  Simulated Generator Controller : Subsystem
  Switch : Switch  Threshold=0.5
  control mode 1 for Woodward 0 for simulation 1 : Constant  Value=control_mode
  A : PMIOPort  Port=1  Side=Right
  B : PMIOPort  Port=2  Side=Right
  C : PMIOPort  Port=3  Side=Right
  tag scope: cntrl_mode=global, gen_m=global
  wires:
  Simulated Generator Controller/1("wref, Vref") -> Switch/3  "simulated"
  Enable_generator/1 -> 60kW Generator with  Primary Controllers/3(Enable)
  60kW Generator with  Primary Controllers/1(m) -> [gen_m]
  Demux/1 -> 60kW Generator with  Primary Controllers/1(wref), Scope/1  "w_ref"
  Demux/2 -> 60kW Generator with  Primary Controllers/2(Vtref), Scope/2  "v_ref"
  Interface between Woodward Controller and simated generator/1(wref,Vref) -> Switch/1
  Switch/1 -> Demux/1
  control mode 1 for Woodward 0 for simulation 1/1 -> [cntrl_mode]
  [cntrl_mode] -> Switch/2
  Woodward Modbus Ref for Governor/1 -> Interface between Woodward Controller and simated generator/1(Woodward for wref)
  Woodward Modbus Ref for AVR/1 -> Interface between Woodward Controller and simated generator/2(Woodward for Vref)
  Woodward meas w/1 -> 60kW Generator with  Primary Controllers/4(w_meas_Woodward)
  Woodward meas V/1 -> 60kW Generator with  Primary Controllers/5(V_meas_Woodward)
  connections:
  A/RConn1 -- 60kW Generator with  Primary Controllers/RConn1
  60kW Generator with  Primary Controllers/RConn2 -- B/RConn1
  C/RConn1 -- 60kW Generator with  Primary Controllers/RConn3

== system HIL_GenSet/GenSet_RTLAB ==
  Bus Selector1 : BusSelector  OutputSignals="Output active power   Peo (pu),Output reactive power  Qeo (pu)"
  Demux : Demux  Outputs=2
  Enable_generator : Constant  Value=enable_gen
  Generator with  Primary Controllers1 : Subsystem
  Multiport Switch : MultiPortSwitch  zeroidx=off
  Mux1 : Mux  Inputs=2
  Mux2 : Mux  Inputs=2
  Mux3 : Mux  Inputs=2
  PQ control : Subsystem
  PV control : Subsystem
  Pref : Constant  Value=set_Pref
  Qref : Constant  Value=set_Qref
  mode (1-3) : Constant  Value=mode
  set_vtref : Constant  Value=set_vref
  set_wref : Constant  Value=set_wref
  A : PMIOPort  Port=1  Side=Right
  B : PMIOPort  Port=2  Side=Right
  C : PMIOPort  Port=3  Side=Right
  tag scope: gen_m=global
  wires:
  Generator with  Primary Controllers1/1(m) -> [gen_m]
  Enable_generator/1 -> Generator with  Primary Controllers1/3(Enable)
  mode (1-3)/1 -> Multiport Switch/1
  Qref/1 -> PQ control/3(Q_ref (pu))
  set_wref/1 -> Mux3/1
  Bus Selector1/2 -> PQ control/4(Q (pu))  "<Output reactive power  Qeo (pu)>"
  Pref/1 -> PV control/1(P_ref (pu)), PQ control/1(P_ref (pu))
  Mux3/1 -> Multiport Switch/4
  Mux2/1 -> Multiport Switch/3
  Mux1/1 -> Multiport Switch/2
  set_vtref/1 -> Mux3/2, Mux2/2
  Demux/2 -> Generator with  Primary Controllers1/2(Vtref)  "v_ref"
  Demux/1 -> Generator with  Primary Controllers1/1(wref)  "w_ref"
  Multiport Switch/1 -> Demux/1
  PV control/1(w_ref (pu)) -> Mux2/1
  PQ control/2(V_ref (pu)) -> Mux1/2
  PQ control/1(w_ref (pu)) -> Mux1/1
  [gen_m] -> Bus Selector1/1
  Bus Selector1/1 -> PV control/2(P (pu)), PQ control/2(P (pu))  "<Output active power   Peo (pu)>"
  connections:
  C/RConn1 -- Generator with  Primary Controllers1/RConn3
  B/RConn1 -- Generator with  Primary Controllers1/RConn2
  A/RConn1 -- Generator with  Primary Controllers1/RConn1

== system HIL_GenSet/GenSet_simOnly ==
  Bus Selector1 : BusSelector  OutputSignals="Output active power   Peo (pu),Output reactive power  Qeo (pu)"
  Demux : Demux  Outputs=2
  Enable_generator : Constant  Value=enable_gen
  Generator with  Primary Controllers1 : Subsystem
  Multiport Switch : MultiPortSwitch  zeroidx=off
  Mux1 : Mux  Inputs=2
  Mux2 : Mux  Inputs=2
  Mux3 : Mux  Inputs=2
  PQ control : Subsystem
  PV control : Subsystem
  Pref : Constant  Value=set_Pref
  Qref : Constant  Value=set_Qref
  mode (1-3) : Constant  Value=mode
  set_vtref : Constant  Value=set_vref
  set_wref : Constant  Value=set_wref
  A : PMIOPort  Port=1  Side=Right
  B : PMIOPort  Port=2  Side=Right
  C : PMIOPort  Port=3  Side=Right
  tag scope: gen_m=global
  wires:
  Generator with  Primary Controllers1/1(m) -> [gen_m]
  Enable_generator/1 -> Generator with  Primary Controllers1/3(Enable)
  mode (1-3)/1 -> Multiport Switch/1
  Qref/1 -> PQ control/3(Q_ref (pu))
  set_wref/1 -> Mux3/1
  Bus Selector1/2 -> PQ control/4(Q (pu))  "<Output reactive power  Qeo (pu)>"
  Pref/1 -> PV control/1(P_ref (pu)), PQ control/1(P_ref (pu))
  Mux3/1 -> Multiport Switch/4
  Mux2/1 -> Multiport Switch/3
  Mux1/1 -> Multiport Switch/2
  set_vtref/1 -> Mux3/2, Mux2/2
  Demux/2 -> Generator with  Primary Controllers1/2(Vtref)  "v_ref"
  Demux/1 -> Generator with  Primary Controllers1/1(wref)  "w_ref"
  Multiport Switch/1 -> Demux/1
  PV control/1(w_ref (pu)) -> Mux2/1
  PQ control/2(V_ref (pu)) -> Mux1/2
  PQ control/1(w_ref (pu)) -> Mux1/1
  [gen_m] -> Bus Selector1/1
  Bus Selector1/1 -> PV control/2(P (pu)), PQ control/2(P (pu))  "<Output active power   Peo (pu)>"
  connections:
  C/RConn1 -- Generator with  Primary Controllers1/RConn3
  B/RConn1 -- Generator with  Primary Controllers1/RConn2
  A/RConn1 -- Generator with  Primary Controllers1/RConn1

== system HIL_GenSet/Gen_3.5MW_external_control ==
  1 - PQ 2 - PV 3 - VF : Constant
  Bus Creator : BusCreator  Inputs=5
  DONOTCHANGE : Constant
  F : simulink/Math Operations/Slider Gain  low=0.97  gain=1  high=1.03
  P : simulink/Math Operations/Slider Gain  low=0  gain=0.8  high=1.1
  Q : simulink/Math Operations/Slider Gain  low=0.01  gain=0.2  high=0.4
  V : simulink/Math Operations/Slider Gain  low=0.9  gain=1  high=1.1
  S : Outport
  wires:
  DONOTCHANGE/1 -> P/1, Q/1, V/1, F/1
  Bus Creator/1 -> S/1
  P/1 -> Bus Creator/1  "P"
  Q/1 -> Bus Creator/2  "Q"
  V/1 -> Bus Creator/3  "V"
  F/1 -> Bus Creator/4  "F"
  1 - PQ 2 - PV 3 - VF/1 -> Bus Creator/5  "Mode"

== system HIL_GenSet/Gen_900kW_external_control ==
  1 - PQ 2 - PV 3 - VF : Constant
  Bus Creator : BusCreator  Inputs=6
  DONOTCHANGE : Constant
  F : simulink/Math Operations/Slider Gain  low=0  gain=1  high=1
  P : simulink/Math Operations/Slider Gain  low=0  gain=0.9  high=1
  Q : simulink/Math Operations/Slider Gain  low=0  gain=0.2  high=0.5
  V : simulink/Math Operations/Slider Gain  low=0  gain=1  high=1
  e : Constant
  S : Outport
  wires:
  1 - PQ 2 - PV 3 - VF/1 -> Bus Creator/5  "Mode"
  F/1 -> Bus Creator/4  "F"
  V/1 -> Bus Creator/3  "V"
  Q/1 -> Bus Creator/2  "Q"
  P/1 -> Bus Creator/1  "P"
  Bus Creator/1 -> S/1
  DONOTCHANGE/1 -> F/1, V/1, Q/1, P/1
  e/1 -> Bus Creator/6  "Enable"

== system HIL_GenSet/GenSet_3p5MW_RTLAB/60kW Generator with  Primary Controllers ==
  note: Mirjana M: Parameters for this generators are preset parameters from SimPower System for 72.5kVAr
  wref : Inport
  Vtref : Inport  Port=2
  Enable : Inport  Port=3
  w_meas_Woodward : Inport  Port=4
  V_meas_Woodward : Inport  Port=5
  72.5 kva Diesel Engine Speed & Voltage Control fast : Subsystem
  Scope2 : Scope  NumInputPorts=2
      settings: YMin=0.949571~0.99979  YMax=1.04953~1  SaveName=ScopeData6
  Synchronous Machine pu Fundamental : powerlib/Machines/Synchronous Machine pu Fundamental  PresetModel=No  MechanicalLoad=Mechanical power Pm  ShowDetailedParameters=on  RotorType=Salient-pole  NominalParameters=[4.375+006 460 60]  Stator=[0.008979 0.05 2.35 1.72]  Field=[0.00206 0.511]  Dampers2=[0.0652, 0.5134, 0.0287, 0.2553, 7.765e-3, 0.9167 ]  Dampers1=[0.2826 3.738 0.02545 0.2392]  Mechanical=[0.3468 0.009238 2]  PolePairs=2  InitialConditions="[ 0  0  0  0  0  0  0  0  0 ]"  SetSaturation=off  Saturation=[0.6404,0.7127,0.8441,0.9214,0.9956,1.082,1.19,1.316,1.457;0.7,0.7698,0.8872,0.9466,0.9969,1.046,1.1,1.151,1.201]  Units=per unit fundamental parameters  LoadFlowParameters=[1,0,0,0,0]  TsPowergui=0  TsBlock=-1  IterativeModel=Forward Euler  BusType=PV  Pref=0  Qref=0  Qmin=-inf  Qmax=inf  PLF=0  QLF=0
  A : PMIOPort  Port=1  Side=Right
  B : PMIOPort  Port=2  Side=Right
  C : PMIOPort  Port=3  Side=Right
  m : Outport
  wires:
  Enable/1 -> 72.5 kva Diesel Engine Speed & Voltage Control fast/3(Generator Enable)
  Vtref/1 -> 72.5 kva Diesel Engine Speed & Voltage Control fast/2(Vtref)
  wref/1 -> 72.5 kva Diesel Engine Speed & Voltage Control fast/1(wref)
  72.5 kva Diesel Engine Speed & Voltage Control fast/3(Vt) -> Scope2/1
  72.5 kva Diesel Engine Speed & Voltage Control fast/4(w) -> Scope2/2
  Synchronous Machine pu Fundamental/1 -> m/1, 72.5 kva Diesel Engine Speed & Voltage Control fast/4(m)
  72.5 kva Diesel Engine Speed & Voltage Control fast/2(Vf) -> Synchronous Machine pu Fundamental/2
  72.5 kva Diesel Engine Speed & Voltage Control fast/1(Pm) -> Synchronous Machine pu Fundamental/1
  w_meas_Woodward/1 -> 72.5 kva Diesel Engine Speed & Voltage Control fast/5(w_meas_Wood)
  V_meas_Woodward/1 -> 72.5 kva Diesel Engine Speed & Voltage Control fast/6(V_meas_Wood)
  connections:
  C/RConn1 -- Synchronous Machine pu Fundamental/RConn3
  B/RConn1 -- Synchronous Machine pu Fundamental/RConn2
  A/RConn1 -- Synchronous Machine pu Fundamental/RConn1

== system HIL_GenSet/GenSet_3p5MW_RTLAB/Interface between Woodward Controller and simated generator ==
  note: Note: This may need a different scaling because it is the reference signal.
      | Reference has to be between 0.95 and 1.05 pu in order to be in tolerance.
  Woodward for wref : Inport
  Woodward for Vref : Inport  Port=2
  Add2 : Sum
  Add3 : Sum
  Gain2 : Gain  Gain=0.005
  Gain3 : Gain  Gain=0.005
  Mux1 : Mux  Inputs=2
  Vref_set : Constant
  wref_set : Constant
  wref,Vref : Outport
  wires:
  Gain2/1 -> Add2/1  "bias"
  Add2/1 -> Mux1/1
  wref_set/1 -> Add2/2
  Gain3/1 -> Add3/1  "bias"
  Vref_set/1 -> Add3/2
  Add3/1 -> Mux1/2
  Woodward for wref/1 -> Gain2/1
  Mux1/1 -> wref,Vref/1  "hardware"
  Woodward for Vref/1 -> Gain3/1

== system HIL_GenSet/GenSet_3p5MW_RTLAB/Simulated Generator Controller ==
  Bus Selector1 : BusSelector  OutputSignals="Output active power   Peo (pu),Output reactive power  Qeo (pu)"
  Multiport Switch : MultiPortSwitch  zeroidx=off
  Mux1 : Mux  Inputs=2
  Mux2 : Mux  Inputs=2
  Mux3 : Mux  Inputs=2
  PQ control : Subsystem
  PV control : Subsystem
  Pref : Constant  Value=set_Pref
  Qref : Constant  Value=set_Qref
  mode (1-3) : Constant  Value=mode
  set_vtref : Constant  Value=set_vref
  set_wref : Constant  Value=set_wref
  "wref, Vref" : Outport
  wires:
  Bus Selector1/1 -> PQ control/2(P (pu)), PV control/2(P (pu))  "<Output active power   Peo (pu)>"
  [gen_m] -> Bus Selector1/1
  PQ control/1(w_ref (pu)) -> Mux1/1
  PQ control/2(V_ref (pu)) -> Mux1/2
  PV control/1(w_ref (pu)) -> Mux2/1
  set_vtref/1 -> Mux2/2, Mux3/2
  Mux1/1 -> Multiport Switch/2
  Mux2/1 -> Multiport Switch/3
  Mux3/1 -> Multiport Switch/4
  Pref/1 -> PQ control/1(P_ref (pu)), PV control/1(P_ref (pu))
  Bus Selector1/2 -> PQ control/4(Q (pu))  "<Output reactive power  Qeo (pu)>"
  set_wref/1 -> Mux3/1
  Qref/1 -> PQ control/3(Q_ref (pu))
  mode (1-3)/1 -> Multiport Switch/1
  Multiport Switch/1 -> "wref, Vref"/1
